simulink library "risingDebounce_ul"  (R2018b)
settings: Solver=VariableStepAuto  StartTime=0.0  StopTime=10.0  RelTol=1e-3
settings Model: Creator=mcobb  LastModifiedBy=mae-ncsucore

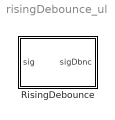
== system risingDebounce_ul ==
  RisingDebounce : Subsystem  mask{threshold=0.5, timeDelay_s=0.1}
      mask prompts: timeDelay_s "Debounce Duration"
      mask Display:
      | str_thres = get_param(gcb,'threshold');
      | str_db = get_param(gcb,'timeDelay_s');
      | 
      | global params;
      | if contains(str_thres,'params')
      | %     dict = Simulink.data.dictionary.open('paramsDataDictionary.sldd');
      | %     sect = getSection(dict,'Design Data');
      | 
      |     str = strsplit(str_thres,'.');
      |     var = getVariable(str{2});
      |     str_thres = num2str(var.Value);
      | 
      | %     var = getEntry(sect,str{1});
      | %     val = getValue(var);
      | %     str_thres = num2str(val.Value);
      | else
      |    str_thres = round(str2num(str_thres),2);
      |    str_thres = num2str(str_thres);
      | end
      | 
      | if contains(str_db,'params')
      |     str = strsplit(str_db,'.');
      |     var = getVariable(str{2});
      |     str_db = num2str(var.Value);
      | 
      | %     var = getEntry(sect,str{1});
      | %     val = getValue(var);
      | %     str_db = num2str(val.Value);
      | %     str_thres = num2str(eval(get_param(gcb,'threshold')));
      | %     str_db = num2str(eval(get_param(gcb,'timeDelay_s')));
      | else
      |    str_db = round(str2num(str_db),2);
      |    str_db = num2str(str_db);
      | end
      | 
      | str = ['Threshold = ' str_thres  '\n ' 'Delay = ' str_db  ];
      |     disp(str)

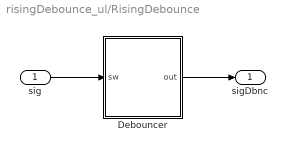
== system risingDebounce_ul/RisingDebounce ==
  sig : Inport
  Debouncer : Stateflow chart  TreatAsAtomicUnit=on
  sigDbnc : Outport
  wires:
  sig/1 -> Debouncer/1(sw)
  Debouncer/1(out) -> sigDbnc/1

== stateflow chart risingDebounce_ul/RisingDebounce/Debouncer ==
  settings: updateMethod=DISCRETE
  state Off
    entry: out = false;
  state On
    entry: out = true;
  (default) -> Off
  On -> Off : [sw < threshold]
  Off -> On : [duration(sw >= threshold) > timeDelay_s ]
  data: sw input; timeDelay_s parameter; threshold parameter; out output
